simulink model "Attitude Stability of tilt-rotor UAV during Obstacle Avoidance and Transition mode"  (R2022a)
settings: Solver=ode45  StartTime=0.0  StopTime=30  RelTol=1e-3
libraries: simulink x1
settings Model: Creator=Ren Mingyu  LastModifiedBy=Ren Mingyu

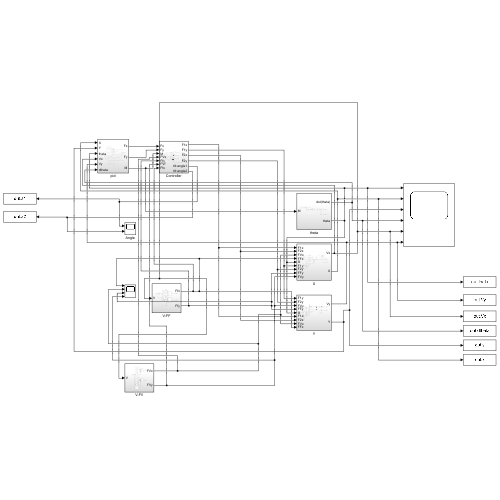
[thumbnail: Simulink's stored preview of the top-level diagram]
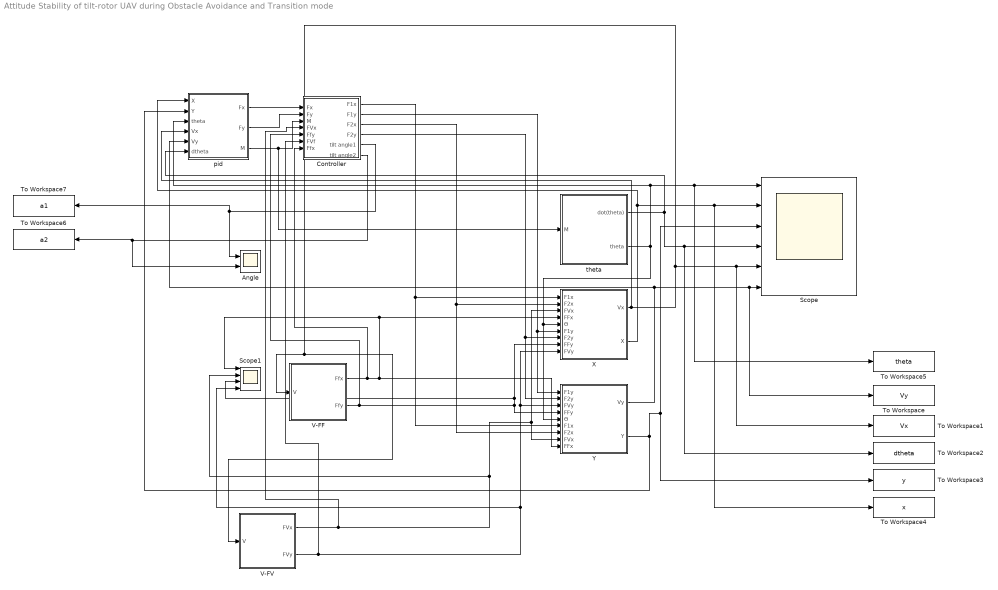
== system Attitude Stability of tilt-rotor UAV during Obstacle Avoidance and Transition mode ==
  Angle : Scope  NumInputPorts=2
  Controller : Subsystem
  Scope : Scope  NumInputPorts=6
  Scope1 : Scope  NumInputPorts=4
  To Workspace : ToWorkspace  VariableName=Vy  SampleTime=-1
      settings: Save2DSignal=2-D array (concatenate along first dimension)
  To Workspace1 : ToWorkspace  VariableName=Vx  SampleTime=-1
      settings: Save2DSignal=2-D array (concatenate along first dimension)
  To Workspace2 : ToWorkspace  VariableName=dtheta  SampleTime=-1
      settings: Save2DSignal=2-D array (concatenate along first dimension)
  To Workspace3 : ToWorkspace  VariableName=y  SaveFormat=Timeseries  SampleTime=-1
  To Workspace4 : ToWorkspace  VariableName=x  SaveFormat=Timeseries  SampleTime=-1
  To Workspace5 : ToWorkspace  VariableName=theta  SampleTime=-1
  To Workspace6 : ToWorkspace  VariableName=a2  SampleTime=-1
      settings: Save2DSignal=2-D array (concatenate along first dimension)
  To Workspace7 : ToWorkspace  VariableName=a1  SampleTime=-1
      settings: Save2DSignal=2-D array (concatenate along first dimension)
  V-FF : Subsystem
  V-FV : Subsystem
  X : Subsystem
  Y : Subsystem
  pid : Subsystem
  theta : Subsystem
  wires:
  V-FV/2(FVy) -> Controller/6(FVf), X/9(FVy), Y/3(FVy), Scope1/4
  V-FV/1(FVx) -> Controller/4(FVx), Y/8(FVx), X/3(FVx), Scope1/2
  Y/2(Y) -> To Workspace3/1, Scope/3, pid/2(Y)
  theta/1(dot(theta)) -> Scope/4, To Workspace2/1, pid/6(dtheta)
  X/1(Vx) -> Scope/5, To Workspace1/1, V-FV/1(V), V-FF/1(V), pid/4(Vx)
  V-FF/1(Ffx) -> Controller/7(Ffx), X/4(FFx), Scope1/1, Y/9(FFx)
  V-FF/2(Ffy) -> Controller/5(Ffy), X/8(FFy), Scope1/3, Y/4(FFy)
  Controller/1(F1x) -> Y/6(F1x), X/1(F1x)
  Controller/2(F1y) -> Y/1(F1y), X/6(F1y)
  Controller/3(F2x) -> Y/7(F2x), X/2(F2x)
  Controller/4(F2y) -> Y/2(F2y), X/7(F2y)
  pid/1(Fx) -> Controller/1(Fx)
  pid/2(Fy) -> Controller/2(Fy)
  pid/3(M) -> theta/1(M), Controller/3(M)
  X/2(X) -> Scope/2, To Workspace4/1, pid/1(X)
  theta/2(theta) -> Y/5(Θ), X/5(Θ), pid/3(theta), Scope/1, To Workspace5/1
  Y/1(Vy) -> To Workspace/1, Scope/6, pid/5(Vy)
  Controller/6(tilt angle2) -> Angle/2, To Workspace6/1
  Controller/5(tilt angle1) -> Angle/1, To Workspace7/1

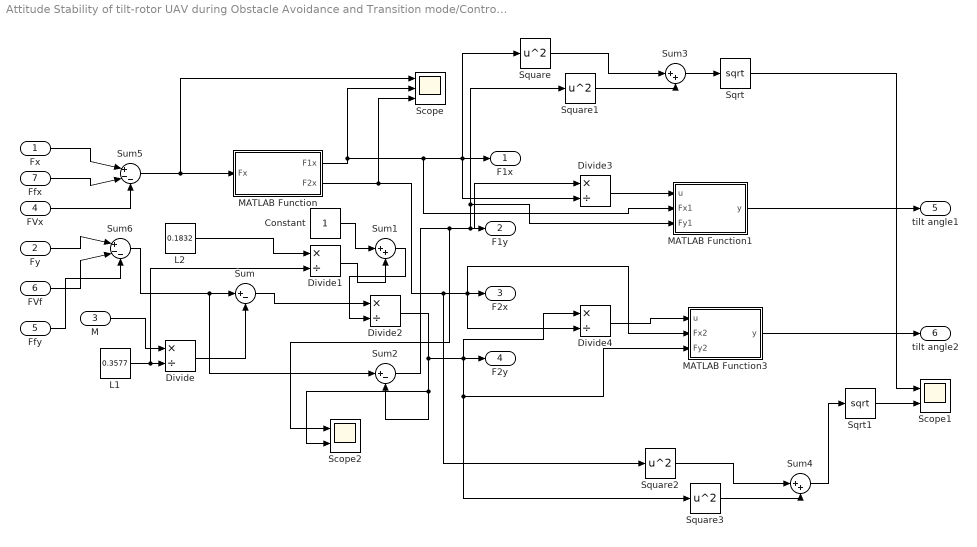
== system Attitude Stability of tilt-rotor UAV during Obstacle Avoidance and Transition mode/Controller ==
  Fx : Inport
  Fy : Inport  Port=2
  M : Inport  Port=3
  FVx : Inport  Port=4
  Ffy : Inport  Port=5
  FVf : Inport  Port=6
  Ffx : Inport  Port=7
  Constant : Constant
  Divide{,1..4} (5 alike) : Product  Inputs=*/
  L1 : Constant  Value=0.3577
  L2 : Constant  Value=0.1832
  MATLAB Function : MATLAB Function  TreatAsAtomicUnit=on
  MATLAB Function1 : MATLAB Function  TreatAsAtomicUnit=on
  MATLAB Function3 : MATLAB Function  TreatAsAtomicUnit=on
  Scope : Scope  NumInputPorts=3
  Scope1 : Scope  NumInputPorts=2
  Scope2 : Scope  NumInputPorts=2
  Sqrt : Sqrt
  Sqrt1 : Sqrt
  Square{,1..3} (4 alike) : Math  Operator=square
  Sum : Sum  Inputs=|+-
  Sum1 : Sum  Inputs=|++
  Sum2 : Sum  Inputs=|+-
  Sum3 : Sum  Inputs=|++
  Sum4 : Sum  Inputs=|++
  Sum5 : Sum  Inputs=|+--
  Sum6 : Sum  Inputs=|+--
  F1x : Outport
  F1y : Outport  Port=2
  F2x : Outport  Port=3
  F2y : Outport  Port=4
  tilt angle1 : Outport  Port=5
  tilt angle2 : Outport  Port=6
  wires:
  M/1 -> Divide/1
  L1/1 -> Divide1/2, Divide/2
  Divide/1 -> Sum/2
  L2/1 -> Divide1/1
  Constant/1 -> Sum1/1
  Divide1/1 -> Sum1/2
  Sum/1 -> Divide2/1
  Sum1/1 -> Divide2/2
  Divide2/1 -> Scope2/2, Sum2/2, MATLAB Function3/3(Fy2), Square3/1, Divide4/1, F2y/1
  Sum2/1 -> Scope2/1, MATLAB Function1/3(Fy1), Square1/1, F1y/1, Divide3/1
  MATLAB Function/1(F1x) -> Scope/2, MATLAB Function1/2(Fx1), Square/1, Divide3/2, F1x/1
  MATLAB Function/2(F2x) -> Scope/3, Square2/1, MATLAB Function3/2(Fx2), Divide4/2, F2x/1
  MATLAB Function1/1(y) -> tilt angle1/1
  MATLAB Function3/1(y) -> tilt angle2/1
  Square/1 -> Sum3/1
  Square1/1 -> Sum3/2
  Sum3/1 -> Sqrt/1
  Sum4/1 -> Sqrt1/1
  Square3/1 -> Sum4/2
  Square2/1 -> Sum4/1
  Sqrt/1 -> Scope1/1
  Sqrt1/1 -> Scope1/2
  Divide3/1 -> MATLAB Function1/1(u)
  Divide4/1 -> MATLAB Function3/1(u)
  Sum5/1 -> Scope/1, MATLAB Function/1(Fx)
  Fx/1 -> Sum5/1
  Ffx/1 -> Sum5/2
  FVx/1 -> Sum5/3
  Sum6/1 -> Sum2/1, Sum/1
  Fy/1 -> Sum6/1
  FVf/1 -> Sum6/2
  Ffy/1 -> Sum6/3

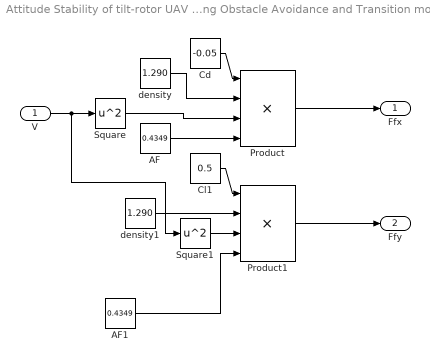
== system Attitude Stability of tilt-rotor UAV during Obstacle Avoidance and Transition mode/V-FF ==
  V : Inport
  AF : Constant  Value=0.4349
  AF1 : Constant  Value=0.4349
  Cd : Constant  Value=-0.05
  Cl1 : Constant  Value=0.5
  Product : Product  Inputs=4
  Product1 : Product  Inputs=4
  Square : Math  Operator=square
  Square1 : Math  Operator=square
  density : Constant  Value=1.290
  density1 : Constant  Value=1.290
  Ffx : Outport
  Ffy : Outport  Port=2
  wires:
  V/1 -> Square1/1, Square/1
  density/1 -> Product/2
  Cd/1 -> Product/1
  Product/1 -> Ffx/1
  density1/1 -> Product1/2
  Cl1/1 -> Product1/1
  Product1/1 -> Ffy/1
  AF1/1 -> Product1/4
  Square1/1 -> Product1/3
  Square/1 -> Product/3
  AF/1 -> Product/4

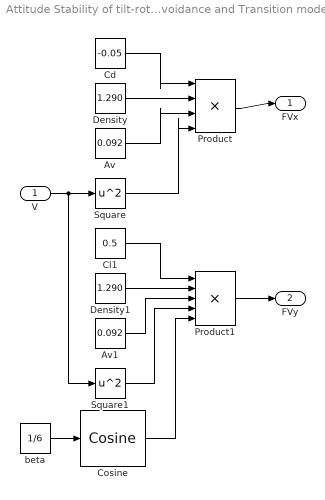
== system Attitude Stability of tilt-rotor UAV during Obstacle Avoidance and Transition mode/V-FV ==
  V : Inport
  Av : Constant  Value=0.092
  Av1 : Constant  Value=0.092
  Cd : Constant  Value=-0.05
  Cl1 : Constant  Value=0.5
  Cosine : simulink/Lookup Tables/Cosine  Formula=cos(2*pi*u)  NumDataPoints=(2^5)+1  OutputWordLength=16  InternalRulePriority=Speed
      settings: SourceProductBaseCode=SL
  Density : Constant  Value=1.290
  Density1 : Constant  Value=1.290
  Product : Product  Inputs=4
  Product1 : Product  Inputs=5
  Square : Math  Operator=square
  Square1 : Math  Operator=square
  beta : Constant  Value=1/6
  FVx : Outport
  FVy : Outport  Port=2
  wires:
  V/1 -> Square1/1, Square/1
  Cd/1 -> Product/1
  Density/1 -> Product/2
  Av/1 -> Product/3
  Square/1 -> Product/4
  Product/1 -> FVx/1
  Square1/1 -> Product1/4
  Density1/1 -> Product1/2
  Cl1/1 -> Product1/1
  Product1/1 -> FVy/1
  Av1/1 -> Product1/3
  beta/1 -> Cosine/1
  Cosine/1 -> Product1/5

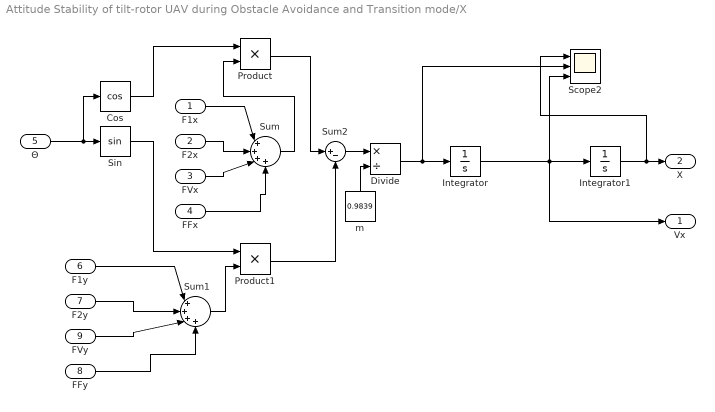
== system Attitude Stability of tilt-rotor UAV during Obstacle Avoidance and Transition mode/X ==
  F1x : Inport
  F2x : Inport  Port=2
  FVx : Inport  Port=3
  FFx : Inport  Port=4
  Θ : Inport  Port=5
  F1y : Inport  Port=6
  F2y : Inport  Port=7
  FFy : Inport  Port=8
  FVy : Inport  Port=9
  Cos : Trigonometry  Operator=cos
  Divide : Product  Inputs=*/
  Integrator : Integrator  InitialCondition=10
  Integrator1 : Integrator
  Product : Product
  Product1 : Product
  Scope2 : Scope  NumInputPorts=3
  Sin : Trigonometry
  Sum : Sum  Inputs=|++++
  Sum1 : Sum  Inputs=|++++
  Sum2 : Sum  Inputs=|+-
  m : Constant  Value=0.9839
  Vx : Outport
  X : Outport  Port=2
  wires:
  m/1 -> Divide/2
  Divide/1 -> Scope2/2, Integrator/1
  Integrator1/1 -> Scope2/1, X/1
  Integrator/1 -> Vx/1, Integrator1/1, Scope2/3
  FVx/1 -> Sum/3
  FFx/1 -> Sum/4
  Θ/1 -> Sin/1, Cos/1
  F1x/1 -> Sum/1
  F2x/1 -> Sum/2
  Sum/1 -> Product/2
  F2y/1 -> Sum1/2
  F1y/1 -> Sum1/1
  FFy/1 -> Sum1/4
  FVy/1 -> Sum1/3
  Sin/1 -> Product1/1
  Sum1/1 -> Product1/2
  Product1/1 -> Sum2/2
  Sum2/1 -> Divide/1
  Cos/1 -> Product/1
  Product/1 -> Sum2/1

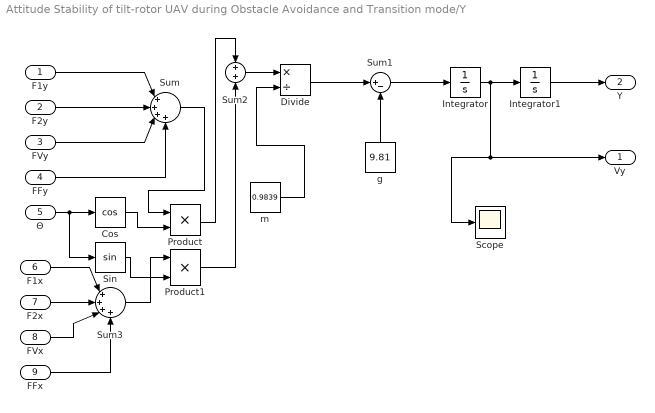
== system Attitude Stability of tilt-rotor UAV during Obstacle Avoidance and Transition mode/Y ==
  F1y : Inport
  F2y : Inport  Port=2
  FVy : Inport  Port=3
  FFy : Inport  Port=4
  Θ : Inport  Port=5
  F1x : Inport  Port=6
  F2x : Inport  Port=7
  FVx : Inport  Port=8
  FFx : Inport  Port=9
  Cos : Trigonometry  Operator=cos
  Divide : Product  Inputs=*/
  Integrator : Integrator
  Integrator1 : Integrator  InitialCondition=5
  Product : Product
  Product1 : Product
  Scope : Scope
  Sin : Trigonometry
  Sum : Sum  Inputs=|++++
  Sum1 : Sum  Inputs=|+-
  Sum2 : Sum
  Sum3 : Sum  Inputs=|++++
  g : Constant  Value=9.81
  m : Constant  Value=0.9839
  Vy : Outport
  Y : Outport  Port=2
  wires:
  m/1 -> Divide/2
  Integrator/1 -> Integrator1/1, Vy/1, Scope/1
  Integrator1/1 -> Y/1
  F2y/1 -> Sum/2
  FVy/1 -> Sum/3
  FFy/1 -> Sum/4
  Divide/1 -> Sum1/1
  Sum1/1 -> Integrator/1
  g/1 -> Sum1/2
  Θ/1 -> Cos/1, Sin/1
  F1y/1 -> Sum/1
  Sum/1 -> Product/1
  Cos/1 -> Product/2
  Sum2/1 -> Divide/1
  Product/1 -> Sum2/1
  Sin/1 -> Product1/2
  Product1/1 -> Sum2/2
  FFx/1 -> Sum3/4
  F1x/1 -> Sum3/1
  F2x/1 -> Sum3/2
  FVx/1 -> Sum3/3
  Sum3/1 -> Product1/1

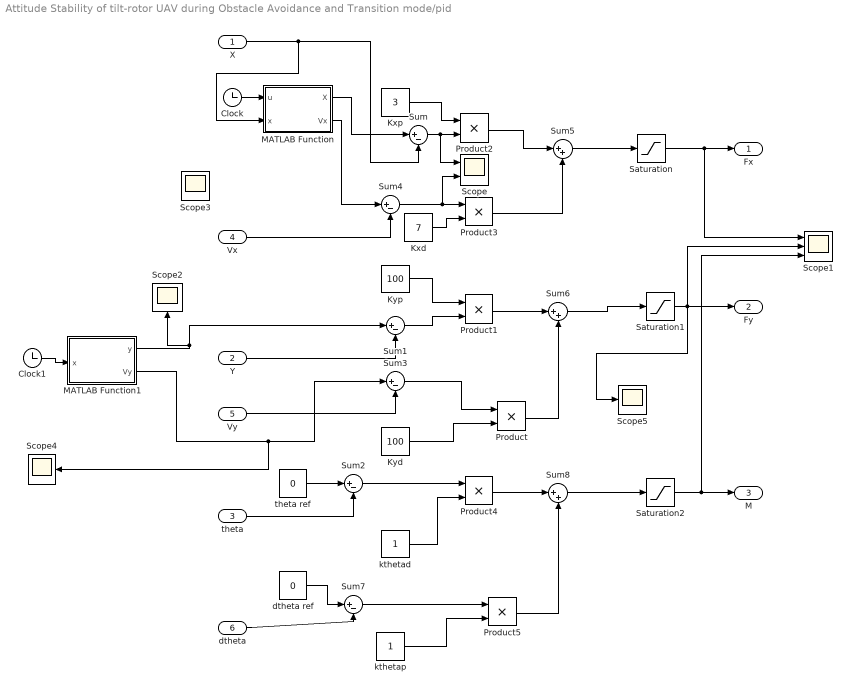
== system Attitude Stability of tilt-rotor UAV during Obstacle Avoidance and Transition mode/pid ==
  X : Inport
  Y : Inport  Port=2
  theta : Inport  Port=3
  Vx : Inport  Port=4
  Vy : Inport  Port=5
  dtheta : Inport  Port=6
  Clock : Clock
  Clock1 : Clock
  Kxd : Constant  Value=7
  Kxp : Constant  Value=3
  Kyd : Constant  Value=100
  Kyp : Constant  Value=100
  MATLAB Function : MATLAB Function  TreatAsAtomicUnit=on
  MATLAB Function1 : MATLAB Function  TreatAsAtomicUnit=on
  Product{,1..5} (6 alike) : Product
  Saturation : Saturate  UpperLimit=1000000000  LowerLimit=-200
  Saturation1 : Saturate  UpperLimit=1000000000  LowerLimit=-200
  Saturation2 : Saturate  UpperLimit=1000000000  LowerLimit=0
  Scope : Scope  NumInputPorts=2
  Scope1 : Scope  NumInputPorts=3
  Scope{2..5} (4 alike) : Scope
  Sum{,1..4,7} (6 alike) : Sum  Inputs=|+-
  Sum5 : Sum  Inputs=|++
  Sum6 : Sum  Inputs=|++
  Sum8 : Sum  Inputs=|++
  dtheta ref : Constant  Value=0
  kthetad : Constant
  kthetap : Constant
  theta ref : Constant  Value=0
  Fx : Outport
  Fy : Outport  Port=2
  M : Outport  Port=3
  wires:
  Y/1 -> Sum1/2
  theta/1 -> Sum2/2
  Vx/1 -> Sum4/2
  Vy/1 -> Sum3/2
  X/1 -> MATLAB Function/2(x), Sum/2
  MATLAB Function1/1(y) -> Sum1/1, Scope2/1
  theta ref/1 -> Sum2/1
  Sum3/1 -> Product/1
  Kyd/1 -> Product/2
  Sum1/1 -> Product1/2
  Kyp/1 -> Product1/1
  Kxp/1 -> Product2/1
  Sum/1 -> Scope/1, Product2/2
  Sum4/1 -> Scope/2, Product3/1
  Kxd/1 -> Product3/2
  Product2/1 -> Sum5/1
  Product3/1 -> Sum5/2
  Sum5/1 -> Saturation/1
  Product1/1 -> Sum6/1
  Product/1 -> Sum6/2
  Sum6/1 -> Saturation1/1
  dtheta ref/1 -> Sum7/1
  dtheta/1 -> Sum7/2
  Sum2/1 -> Product4/1
  kthetad/1 -> Product4/2
  Product4/1 -> Sum8/1
  kthetap/1 -> Product5/2
  Sum7/1 -> Product5/1
  Product5/1 -> Sum8/2
  Sum8/1 -> Saturation2/1
  Saturation/1 -> Scope1/1, Fx/1
  Saturation1/1 -> Scope1/2, Scope5/1, Fy/1
  Saturation2/1 -> Scope1/3, M/1
  Clock1/1 -> MATLAB Function1/1(x)
  MATLAB Function/1(X) -> Sum/1
  MATLAB Function1/2(Vy) -> Sum3/1, Scope4/1
  Clock/1 -> MATLAB Function/1(u)
  MATLAB Function/2(Vx) -> Sum4/1

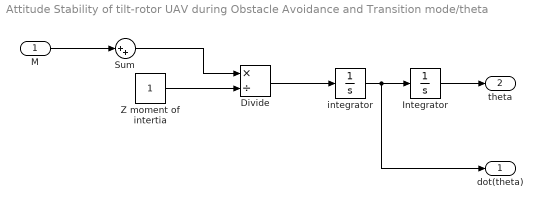
== system Attitude Stability of tilt-rotor UAV during Obstacle Avoidance and Transition mode/theta ==
  M : Inport
  Divide : Product  Inputs=*/
  Integrator : Integrator
  Sum : Sum  Inputs=|++
  Z moment of intertia : Constant
  integrator : Integrator
  dot(theta) : Outport
  theta : Outport  Port=2
  wires:
  Z moment of intertia/1 -> Divide/2
  Divide/1 -> integrator/1
  integrator/1 -> dot(theta)/1, Integrator/1
  Integrator/1 -> theta/1
  M/1 -> Sum/1
  Sum/1 -> Divide/1

== matlab function Attitude Stability of tilt-rotor UAV during Obstacle Avoidance and Transition mode/Controller/MATLAB Function ==
  data: Fx input; F1x output; F2x output
function [F1x, F2x] = solveQP(Fx)
    % 定义目标函数
    fun = @(x) x(1)^2 + x(2)^2;

    % 定义等式约束
    Aeq = [1, 1];
    beq = Fx;

    % 定义不等式约束
    nonlcon = @(x) deal(x(1)^2 + x(2)^2 - 200, []);

    % 定义变量的下界
    lb = [-200, -200];

    % 定义初始点
    x0 = [Fx/2; Fx/2];

    % 定义选项
    options = optimoptions('fmincon','Algorithm','sqp');

    % 调用fmincon函数求解优化问题
    x = fmincon(fun, x0, [], [], Aeq, beq, lb, [], nonlcon, options);

    % 提取解
    F1x = x(1);
    F2x = x(2);
end

== matlab function Attitude Stability of tilt-rotor UAV during Obstacle Avoidance and Transition mode/pid/MATLAB Function ==
  data: u input; X output; Vx output; x input
function [X,Vx] = fcn(u,x)
if u<=20
    X = u;
    Vx=1;
elseif 20<u && u<=25
    Vx=1-(u-20)/5;
    X=x;
else 
    Vx=0;
    X=x;
end

== matlab function Attitude Stability of tilt-rotor UAV during Obstacle Avoidance and Transition mode/Controller/MATLAB Function1 ==
  data: u input; y output; Fx1 input; Fy1 input
function y = fcn(u,Fx1,Fy1)
if Fx1>=0 && Fy1>=0
    y=atan(u)*180/pi;
elseif Fx1<=0 && Fy1>=0
    y=atan(u)*180/pi+180;
elseif Fx1<=0 && Fy1<=0
    y=atan(u)*180/pi+180;
else
    y=atan(u)*180/pi;
end

== matlab function Attitude Stability of tilt-rotor UAV during Obstacle Avoidance and Transition mode/pid/MATLAB Function1 ==
  data: x input; y output; Vy output
function [y,Vy] = fcn(x)
if x<=20
a0  =  7.5087;  
a1=-2.1673;
b1  =  4.7392;   
a2   = -0.2270 ;   
b2  =  -0.5158 ;  
a3  =  0.1598  ;  
b3  =  -0.3852  ;  
a4  =  0.1270  ;  
b4  =  0.2219  ;   
a5  =  -0.2227 ;   
b5  =  0.0365 ;    
w  =   0.3127  ;

y = a0 + a1*cos(x*w) + b1*sin(x*w) + a2*cos(2*x*w) + b2*sin(2*x*w) + a3*cos(3*x*w) + b3*sin(3*x*w) + a4*cos(4*x*w) + b4*sin(4*x*w) + a5*cos(5*x*w) + b5*sin(5*x*w);
Vy= -w*a1*sin(x*w) + w*b1*cos(x*w) - 2*w*a2*sin(2*x*w) + 2*w*b2*cos(2*x*w) -3*w* a3*sin(3*x*w) + 3*w*b3*cos(3*x*w) -4*w*a4*sin(4*x*w) + 4*w*b4*cos(4*x*w) -5*w*a5*sin(5*x*w) + 5*w*b5*cos(5*x*w);
elseif 20<x && x<=25.075
    y=5.075-(x-20);
    Vy=1;
else 
    y=0;
    Vy=1-1*(x-25.075)/4.925;
end

== matlab function Attitude Stability of tilt-rotor UAV during Obstacle Avoidance and Transition mode/Controller/MATLAB Function3 ==
  data: u input; y output; Fx2 input; Fy2 input
function y = fcn(u,Fx2,Fy2)
if Fx2>=0 && Fy2>=0
    y=atan(u)*180/pi;
elseif Fx2<=0 && Fy2>=0
    y=atan(u)*180/pi+180;
elseif Fx2<=0 && Fy2<=0
    y=atan(u)*180/pi+180;
else
    y=atan(u)*180/pi;
end
